simulink model "lego_selfbalance_remote"  (R2013b)
settings: Solver=ode3  SolverMode=SingleTasking  StartTime=0.0  StopTime=10.0  RelTol=1e-3
undefined symbols (not defined in the file or in its folder): Speed, Turn
libraries: legonxtlib x7
settings Model: ExtModeTrigDuration=2  Creator=Alphonso Monk  LastModifiedBy=Alphonso Monk
settings OptimizationCC: OptimizeModelRefInitCode=on  LifeSpan=1
settings DebuggingCC: SolverPrmCheckMsg=none
settings HardwareCC: ProdLargestAtomicInteger=Long  ProdLargestAtomicFloat=Float  ProdEndianess=LittleEndian  ProdHWDeviceType=ARM Compatible->ARM 7
settings RTWCC: SystemTargetFile=realtime.tlc  GenerateMakefile=off  TemplateMakefile=realtime.tmf  Description=Run on Target Hardware  RTWVerbose=off  ProcessScript=realtime_make_rtw_hook
settings STFCustomTargetCC: TargetLibSuffix=.a  GenerateSampleERTMain=on  ERTCustomFileBanners=on  SupportNonInlinedSFcns=off  SupportVariableSizeSignals=on  MATLABClassNameForMDSCustomization=Simulink.SoftwareTarget.ERTCustomization  GRTInterface=off  SystemTargetFile=realtime.tlc
settings ERTTargetCC: CodeReplacementLibrary=ANSI_C  GenerateSampleERTMain=on  ParMdlRefBuildCompliant=off  CompOptLevelCompliant=off  ConcurrentExecutionCompliant=off  CombineOutputUpdateFcns=off  ERTFirstTimeCompliant=off  SupportContinuousTime=on  SupportVariableSizeSignals=on  ModelStepFunctionPrototypeControlCompliant=off  CPPClassGenCompliant=off  InlinedParameterPlacement=NonHierarchical  ERTSrcFileBannerTemplate=realtime_code_template.cgt  ERTHdrFileBannerTemplate=realtime_code_template.cgt  ERTDataSrcFileTemplate=realtime_code_template.cgt  ERTDataHdrFileTemplate=realtime_code_template.cgt  ERTCustomFileTemplate=realtime_file_process.tlc

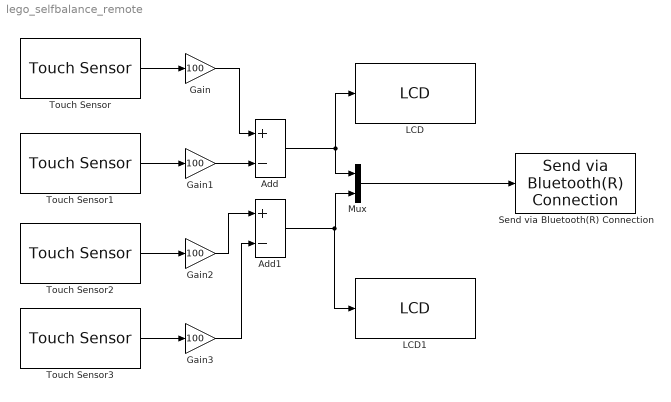
== system lego_selfbalance_remote ==
  Add : Sum  Inputs=+-
  Add1 : Sum  Inputs=+-
  Gain{,1..3} (4 alike) : Gain  Gain=100  OutDataTypeStr=int32
  LCD : legonxtlib/LCD  slcdStr=Speed:  slcdLine=1  slcdFormat=Decimal
  LCD1 : legonxtlib/LCD  slcdStr=Turn:  slcdLine=2  slcdFormat=Decimal
  Mux : Mux  Inputs=2
  Send via Bluetooth(R) Connection : legonxtlib/Send via Bluetooth(R) Connection  mailbox=1
  Touch Sensor : legonxtlib/Touch Sensor  portNumber=2  sampleTime=0.048
  Touch Sensor1 : legonxtlib/Touch Sensor  portNumber=3  sampleTime=0.048
  Touch Sensor2 : legonxtlib/Touch Sensor  portNumber=1  sampleTime=0.048
  Touch Sensor3 : legonxtlib/Touch Sensor  portNumber=4  sampleTime=0.048
  wires:
  Touch Sensor/1 -> Gain/1
  Touch Sensor3/1 -> Gain3/1
  Touch Sensor2/1 -> Gain2/1
  Touch Sensor1/1 -> Gain1/1
  Gain/1 -> Add/1
  Gain1/1 -> Add/2
  Gain2/1 -> Add1/1
  Gain3/1 -> Add1/2
  Add/1 -> Mux/1, LCD/1
  Add1/1 -> LCD1/1, Mux/2
  Mux/1 -> Send via Bluetooth(R) Connection/1
